simulink model "am"  (R2023b)
settings: Solver=FixedStepAuto  StartTime=0.0  StopTime=0.5  FixedStep=1e-5  MaxStep=0.0001  RelTol=1e-4
libraries: simulink x1
settings Model: Creator=B03-304  LastModifiedBy=B03-304

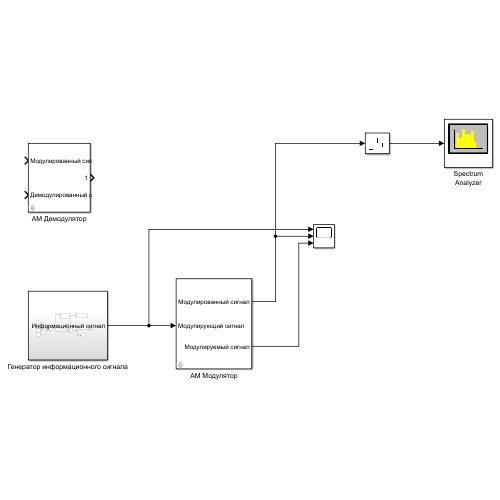
[thumbnail: Simulink's stored preview of the top-level diagram]
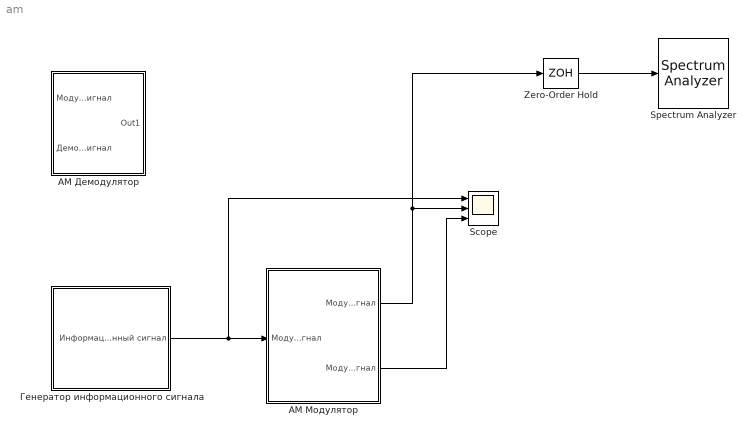
== system am ==
  AM Демодулятор : Subsystem  mask{f0=300, m=0.7}
      mask prompts: f0 "Частота несущей"; m "Порядок модуляции"
  AM Модулятор : Subsystem  mask{f0=300, m=0.5}
      mask prompts: f0 "Частота несущей"; m "Порядок модуляции"
  Scope : Scope  NumInputPorts=3
  Spectrum Analyzer : SpectrumAnalyzer  Tag=simrfV2util1/Spectrum Analyzer  WindowPosition=[560.000000,350.000000,800.000000,500.000000,]  ScopeFrameLocation=window  Method=Welch  PlotAsTwoSidedSpectrum=off  AveragingMethod=Exponential  YLimits=[-197.78046027,48.57882217]
  Zero-Order Hold : ZeroOrderHold  SampleTime=0.0001
  Генератор информационного сигнала : Subsystem
  wires:
  Генератор информационного сигнала/1(Информационный сигнал) -> Scope/1, AM Модулятор/1(Модулирующий сигнал)
  AM Модулятор/1(Модулированный сигнал) -> Zero-Order Hold/1, Scope/2
  AM Модулятор/2(Модулируемый сигнал) -> Scope/3
  Zero-Order Hold/1 -> Spectrum Analyzer/1

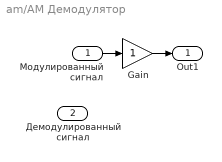
== system am/AM Демодулятор ==
  Модулированный сигнал : Inport
  Демодулированный сигнал : Inport  Port=2
  Gain : Gain
  Out1 : Outport
  wires:
  Модулированный сигнал/1 -> Gain/1
  Gain/1 -> Out1/1

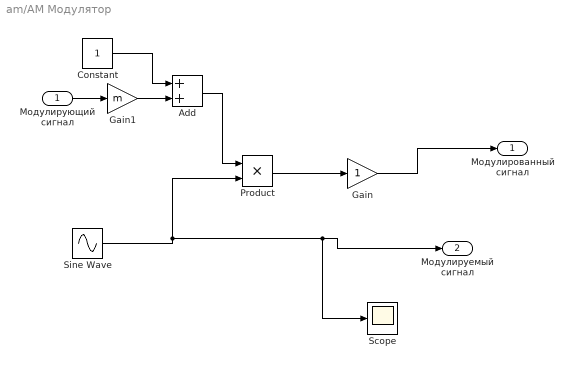
== system am/AM Модулятор ==
  Модулирующий сигнал : Inport
  Add : Sum
  Constant : Constant
  Gain : Gain
  Gain1 : Gain  Gain=m
  Product : Product
  Scope : Scope
  Sine Wave : Sin  Frequency=f0*2*pi  SampleTime=0
  Модулированный сигнал : Outport
  Модулируемый сигнал : Outport  Port=2
  wires:
  Gain/1 -> Модулированный сигнал/1
  Sine Wave/1 -> Product/2, Scope/1, Модулируемый сигнал/1
  Constant/1 -> Add/1
  Модулирующий сигнал/1 -> Gain1/1
  Gain1/1 -> Add/2
  Add/1 -> Product/1
  Product/1 -> Gain/1

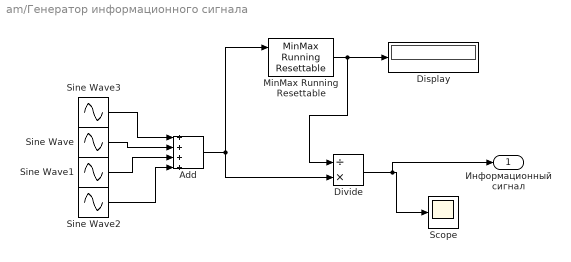
== system am/Генератор информационного сигнала ==
  Add : Sum  Inputs=++++
  Display : Display
  Divide : Product  Inputs=/*
  MinMax Running Resettable : simulink/Math Operations/MinMax Running Resettable  Function=max  vinit=0.1
  Scope : Scope
  Sine Wave : Sin  Frequency=80*2*pi  SampleTime=0
  Sine Wave1 : Sin  Frequency=60*2*pi  SampleTime=0
  Sine Wave2 : Sin  Frequency=40*2*pi  SampleTime=0
  Sine Wave3 : Sin  Frequency=100*2*pi  SampleTime=0
  Информационный сигнал : Outport
  wires:
  Sine Wave3/1 -> Add/1
  Sine Wave/1 -> Add/2
  Sine Wave1/1 -> Add/3
  Sine Wave2/1 -> Add/4
  Add/1 -> MinMax Running Resettable/1, Divide/2
  MinMax Running Resettable/1 -> Divide/1, Display/1
  Divide/1 -> Информационный сигнал/1, Scope/1
